simulink model "meandr_model"  (R2024a)
settings: Solver=FixedStepAuto  StartTime=0.0  StopTime=15  FixedStep=0.0001  RelTol=1e-3
values from neighbouring files (symbols this model uses):
  A = [11 -2 13; 6 -1 6; -6 -1 -8]    [comp_sost.m]    (also in meandr.m = [0 1; 0 0]; out.m; out_copy.m; rank_extended.m)
  B = [2; 0; 0]    [comp_sost.m]    (also in meandr.m = [0; 1]; out.m; out_copy.m; slezh_sost.m)
  C = [1 0]    [meandr.m]    (also in out.m = [2 -2 1]; out_copy.m = [2 -2 1]; rank_extended.m = [2 -2 1])
  Cz = [-2 3 -1]    [comp_sost.m]    (also in meandr.m = -C; out.m; out_copy.m = C; slezh_sost.m)
  Dz = 16/pi * [1 0 1/3 0 1/5 0]    [meandr.m]    (also in out.m = [3 4 2 -3]; out_copy.m = D; slezh_sost.m = [3 4 2 -3])
  G = [35 56 22 -42; -11 -17 -7 12; -6 -10 -5 10; 11 18 6 -13]    [comp_sost.m]    (also in meandr.m = [0 1 0 0 0 0; -1 0 0 0 0 0; 0 0 0 3 0 0; 0 0 -3 0 0 0; 0 0 0; out.m; out_copy.m; rank_extended.m)
  K1 = -inv(R)*B'*P    [comp_sost.m]    (also in meandr.m; out.m = -R\B'*P; out_copy.m; slezh_sost.m)
  K2 = double(Y_sol - K1*P_sol)    [comp_sost.m]    (also in meandr.m; out.m; out_copy.m; slezh_sost.m)
  w0 = [0; 1; 0; 1; 0; 1]    [meandr.m]
  x0 = [1; 1; 1]    [comp_sost.m]    (also in meandr.m = [0; 0])
settings Model: Creator=ventus  LastModifiedBy=ventus

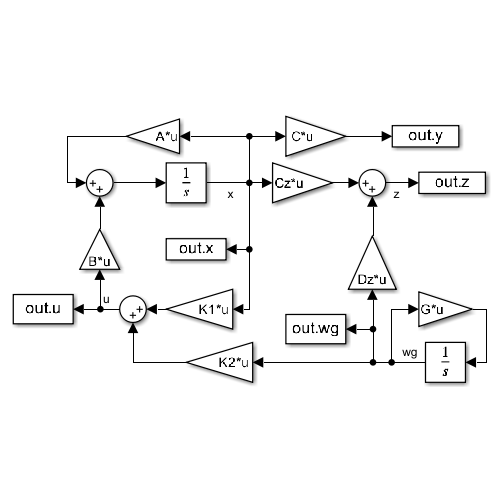
[thumbnail: Simulink's stored preview of the top-level diagram]
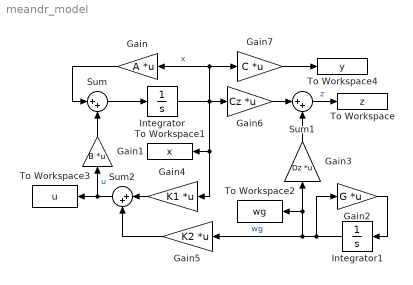
== system meandr_model ==
  Gain : Gain  Gain=A  Multiplication=Matrix(K*u)
  Gain1 : Gain  Gain=B  Multiplication=Matrix(K*u)
  Gain2 : Gain  Gain=G  Multiplication=Matrix(K*u)
  Gain3 : Gain  Gain=Dz  Multiplication=Matrix(K*u)
  Gain4 : Gain  Gain=K1  Multiplication=Matrix(K*u)
  Gain5 : Gain  Gain=K2  Multiplication=Matrix(K*u)
  Gain6 : Gain  Gain=Cz  Multiplication=Matrix(K*u)
  Gain7 : Gain  Gain=C  Multiplication=Matrix(K*u)
  Integrator : Integrator  InitialCondition=x0
  Integrator1 : Integrator  InitialCondition=w0
  Sum : Sum  Inputs=|++
  Sum1 : Sum  Inputs=|++
  Sum2 : Sum  Inputs=|++
  To Workspace : ToWorkspace  VariableName=z  SaveFormat=Timeseries  SampleTime=-1
  To Workspace1 : ToWorkspace  VariableName=x  SaveFormat=Timeseries  SampleTime=-1
  To Workspace2 : ToWorkspace  VariableName=wg  SaveFormat=Timeseries  SampleTime=-1
  To Workspace3 : ToWorkspace  VariableName=u  SaveFormat=Timeseries  SampleTime=-1
  To Workspace4 : ToWorkspace  VariableName=y  SaveFormat=Timeseries  SampleTime=-1
  wires:
  Gain/1 -> Sum/1
  Sum2/1 -> Gain1/1, To Workspace3/1  "u"
  Sum1/1 -> To Workspace/1  "z"
  Gain1/1 -> Sum/2
  Gain2/1 -> Integrator1/1
  Sum/1 -> Integrator/1
  Integrator/1 -> Gain6/1, Gain7/1, Gain/1, Gain4/1, To Workspace1/1  "x"
  Gain6/1 -> Sum1/1
  Gain3/1 -> Sum1/2
  Integrator1/1 -> Gain2/1, To Workspace2/1, Gain3/1, Gain5/1  "wg"
  Gain4/1 -> Sum2/1
  Gain5/1 -> Sum2/2
  Gain7/1 -> To Workspace4/1
